simulink model "filtrage_Simulink__Transfert_Function"  (R2019b)
settings: Solver=VariableStepAuto  StartTime=0.0  StopTime=10.0  RelTol=1e-3
InitFcn:
  | load filtrage_pb_ordre_1.mat;
settings Model: Creator=ivanl  LastModifiedBy=ivanl

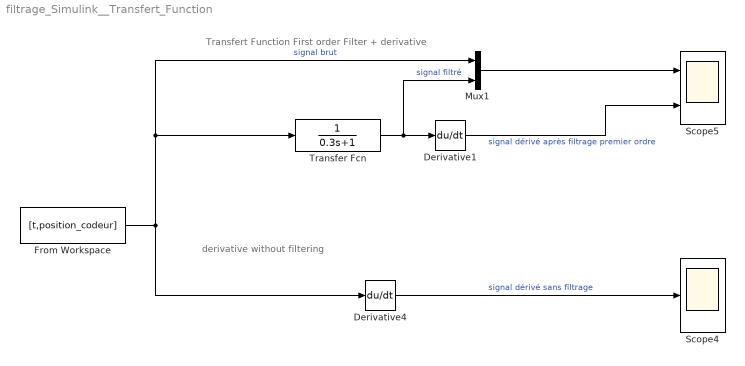
== system filtrage_Simulink__Transfert_Function ==
  note: derivative without filtering
  note: Transfert Function First order Filter + derivative
  Derivative1 : Derivative
  Derivative4 : Derivative
  From Workspace : FromWorkspace  VariableName=[t,position_codeur]  SampleTime=0.001
  Mux1 : Mux  Inputs=2
  Scope4 : Scope
  Scope5 : Scope  NumInputPorts=2
  Transfer Fcn : TransferFcn  Denominator=[0.3 1]
  wires:
  Transfer Fcn/1 -> Mux1/2, Derivative1/1  "signal filtré"
  Mux1/1 -> Scope5/1
  Derivative1/1 -> Scope5/2  "signal dérivé après filtrage premier ordre"
  Derivative4/1 -> Scope4/1  "signal dérivé sans filtrage"
  From Workspace/1 -> Derivative4/1, Transfer Fcn/1, Mux1/1  "signal brut"
